simulink model "Test_DLE"  (R2017b)
settings: Solver=VariableStepAuto  StartTime=0.0  StopTime=100  RelTol=1e-3
settings Model: Creator=ali.safaei  LastModifiedBy=ali.safaei

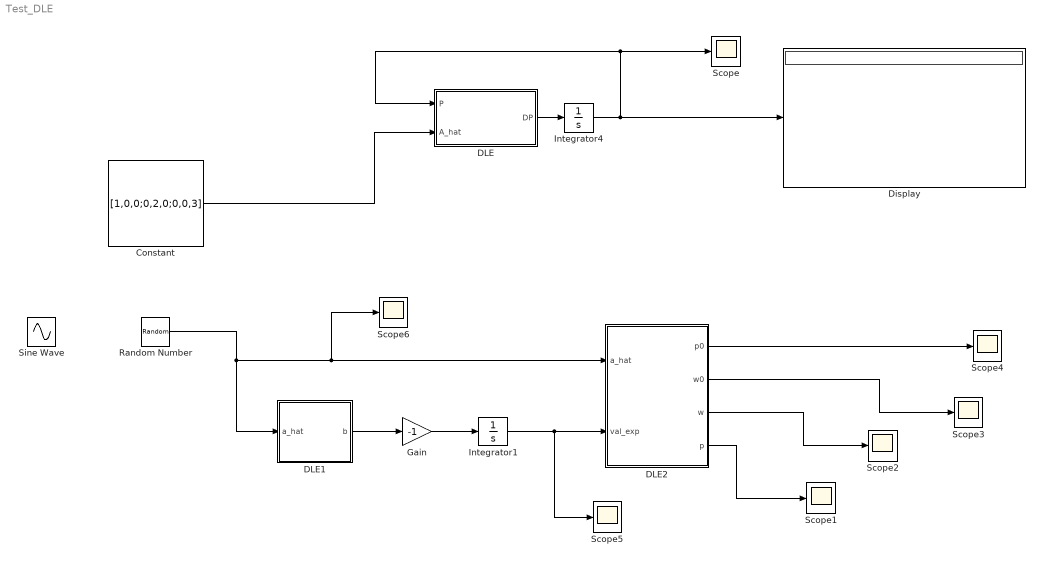
== system Test_DLE ==
  Constant : Constant  Value=[1,0,0;0,2,0;0,0,3]
  DLE : MATLAB Function  TreatAsAtomicUnit=on
  DLE1 : MATLAB Function  TreatAsAtomicUnit=on
  DLE2 : MATLAB Function  TreatAsAtomicUnit=on
  Display : Display
  Gain : Gain  Gain=-1
  Integrator1 : Integrator
  Integrator4 : Integrator  InitialCondition=eye(3)
  Random Number : RandomNumber  SampleTime=0.1
  Scope{,1..6} (7 alike) : Scope
  Sine Wave : Sin  Amplitude=10  Bias=-40  SampleTime=0
  wires:
  DLE/1(DP) -> Integrator4/1
  Integrator4/1 -> Display/1, Scope/1, DLE/1(P)
  Constant/1 -> DLE/2(A_hat)
  DLE1/1(b) -> Gain/1
  Integrator1/1 -> Scope5/1, DLE2/2(val_exp)
  Gain/1 -> Integrator1/1
  DLE2/4(p) -> Scope1/1
  Random Number/1 -> Scope6/1, DLE2/1(a_hat), DLE1/1(a_hat)
  DLE2/3(w) -> Scope2/1
  DLE2/2(w0) -> Scope3/1
  DLE2/1(p0) -> Scope4/1

== matlab function Test_DLE/DLE1 ==
  data: a_hat input; b output
function b = fcn(a_hat)

h = 2;
q = 1e2;
Delta = (a_hat^2) + (2*q*h);
b = 2*sqrt(Delta);

end

== matlab function Test_DLE/DLE2 ==
  data: p0 output; w0 output; w output; a_hat input; p output; val_exp input
function [p0,w0,w,p] = fcn(a_hat,val_exp)

h = 2;
q = 1e+2;
Delta = (a_hat^2) + (2*q*h);
p_init = 1;
p0 = (1/h) * (a_hat - sqrt(Delta));
w0 = 1 / (p_init - p0);
b = 2*sqrt(Delta);
w = (h/b) + (w0 - (h/b))*exp(val_exp);
p = p0 + (1/w);

end

== matlab function Test_DLE/DLE ==
  data: P input; A_hat input; DP output
function DP = fcn(P,A_hat)

Q = 1.0e-0*eye(3);
R = 1.0e+0*eye(3);
h = 2;
DP = - (A_hat*P + P*A_hat') - 2*Q + h*(P'*R*P);

end
